simulink model "resettableTimer_th"  (R2018a)
settings: Solver=FixedStepAuto  StartTime=0.0  StopTime=10.0  FixedStep=sm.Ts  RelTol=1e-3
libraries: resettableTimer x1
settings Model: Creator=mitch  LastModifiedBy=mitch

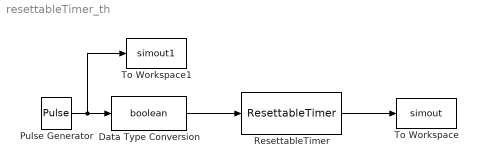
== system resettableTimer_th ==
  Data Type Conversion : DataTypeConversion  OutDataTypeStr=boolean
  Pulse Generator : DiscretePulseGenerator  Period=1000  PulseWidth=750  SampleTime=sm.Ts
  ResettableTimer : resettableTimer/ResettableTimer
  To Workspace : ToWorkspace  VariableName=simout  SaveFormat=Timeseries  SampleTime=-1
  To Workspace1 : ToWorkspace  VariableName=simout1  SaveFormat=Timeseries  SampleTime=-1
  wires:
  ResettableTimer/1 -> To Workspace/1
  Data Type Conversion/1 -> ResettableTimer/1
  Pulse Generator/1 -> To Workspace1/1, Data Type Conversion/1
